simulink model "wtLinModelSimulink_LQI_V6_2021a"  (R2021a)
settings: Solver=FixedStepAuto  StartTime=0.0  StopTime=1000  FixedStep=1/25  RelTol=1e-3
values from neighbouring files (symbols this model uses):
  Alqi = [Alqr		zeros(3,1) ... (first row only)    [wtLin_V164_8MW_V6_LQI.m]
  Alqi_d = sysINT_d.A    [wtLin_V164_8MW_V6_LQI.m]
  Alqr = sysNoFLC2.A    [wtLin_V164_8MW_V6_LQI.m]
  Asys = sys.full.A    [wtLin_V164_8MW_V6_LQI.m]
  Asys_d = sys_d.A    [wtLin_V164_8MW_V6_LQI.m]
  Bdlqi = [Bdlqr; 0]    [wtLin_V164_8MW_V6_LQI.m]
  Bdlqi_d = sysINT_d.B(:,distIndex)    [wtLin_V164_8MW_V6_LQI.m]
  Bdlqr = Blqr(:, distIndex)    [wtLin_V164_8MW_V6_LQI.m]
  Bsys = sys.full.B    [wtLin_V164_8MW_V6_LQI.m]
  Bsys_d = sys_d.B    [wtLin_V164_8MW_V6_LQI.m]
  Bulqi = [Bulqr; 0]    [wtLin_V164_8MW_V6_LQI.m]
  Bulqi_d = sysINT_d.B(:,distIndex+1:end)    [wtLin_V164_8MW_V6_LQI.m]
  Bulqr = Blqr(:, distIndex+1:end)    [wtLin_V164_8MW_V6_LQI.m]
  Clqi = [Clqr	zeros(3,1)]    [wtLin_V164_8MW_V6_LQI.m]
  Clqr = sysNoFLC2.C    [wtLin_V164_8MW_V6_LQI.m]
  Csys = sys.full.C    [wtLin_V164_8MW_V6_LQI.m]
  Csys_d = sys_d.C    [wtLin_V164_8MW_V6_LQI.m]
  opWindSpeed = 16    [wtLin_V164_8MW_V6_LQI.m]
  u_op = [simulationData(1,senIdx.Vhfree); simulationData(1,senIdx.pnt413); simulationData(1,senIdx.pfo017)]    [wtLin_V164_8MW_V6_LQI.m]
  x_bar_init = [py_init vy_init W_init]'    [wtLin_V164_8MW_V6_LQI.m]
  x_bar_init_flc = [0 py_init vy_init W_init]'    [wtLin_V164_8MW_V6_LQI.m]
  x_bar_init_lqi = [py_init vy_init W_init 0]'    [wtLin_V164_8MW_V6_LQI.m]
  x_op_temp = [py_op vy_op W_op]'    [wtLin_V164_8MW_V6_LQI.m]
  x_op_temp_flc = [0 py_op vy_op W_op]'    [wtLin_V164_8MW_V6_LQI.m]
  x_op_temp_lqi = [ py_op vy_op W_op 0]'    [wtLin_V164_8MW_V6_LQI.m]
undefined symbols (not defined in the file or in its folder): Klqi, Klqi_d, Klqr2
settings Model: Creator=martin  LastModifiedBy=MROTR
settings DataIOCC: ExternalInput=tt_vfree  LoadExternalInput=on

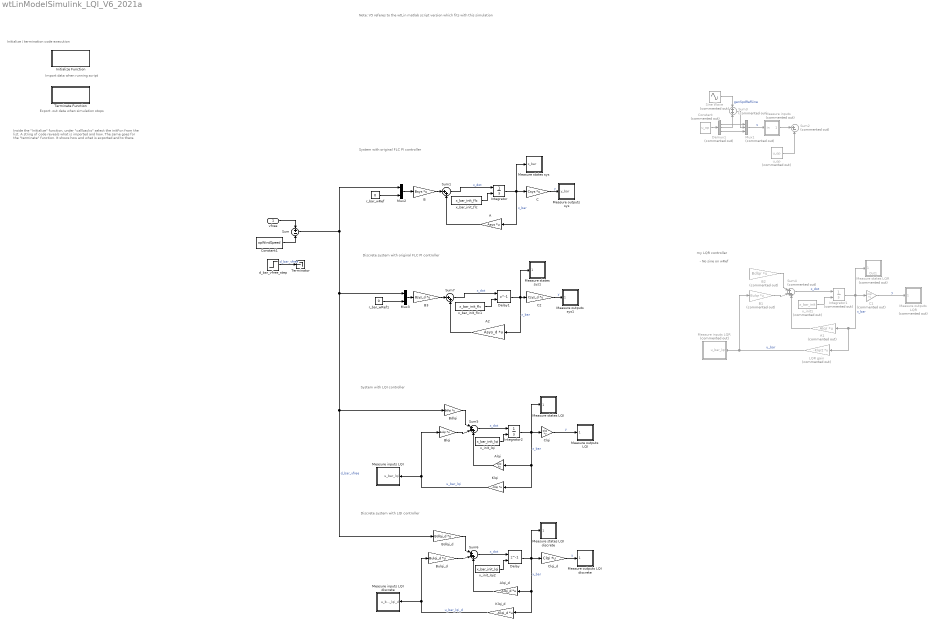
== system wtLinModelSimulink_LQI_V6_2021a ==
  note: Inside the "Initialize" function, under "callbacks" select the initFcn from the list. A string of code reveals what is imported and how.
      | The same goes for the "terminate" function. It shows how and what is exported and to there.
  note: Export .out data when simulation stops
  note: Import data when running script
  note: Initialize / termination code execution
  note: Note: V5 referes to the wtLin matlab script version which fits with this simulation
  note: System with LQI controller
  note: - No sine on wRef
  note: my LQR controller
  note: System with original FLC PI controller
  note: Discrete system with LQI controller
  note: Discrete system with original FLC PI controller
  vfree : Inport
  A : Gain  Gain=Asys  Multiplication=Matrix(K*u)
  A1 : Gain  Commented=on  Gain=Alqr  Multiplication=Matrix(K*u)
  A2 : Gain  Gain=Asys_d  Multiplication=Matrix(K*u)
  Alqi : Gain  Gain=Alqi  Multiplication=Matrix(K*u)
  Alqi_d : Gain  Gain=Alqi_d  Multiplication=Matrix(K*u)
  B : Gain  Gain=Bsys  Multiplication=Matrix(K*u)
  B1 : Gain  Commented=on  Gain=Bulqr  Multiplication=Matrix(K*u)
  B2 : Gain  Commented=on  Gain=Bdlqr  Multiplication=Matrix(K*u)
  B3 : Gain  Gain=Bsys_d  Multiplication=Matrix(K*u)
  Bdlqi : Gain  Gain=Bdlqi  Multiplication=Matrix(K*u)
  Bdlqi_d : Gain  Gain=Bdlqi_d  Multiplication=Matrix(K*u)
  Blqi : Gain  Gain=Bulqi  Multiplication=Matrix(K*u)
  Bulqi_d : Gain  Gain=Bulqi_d  Multiplication=Matrix(K*u)
  C : Gain  Gain=Csys  Multiplication=Matrix(K*u)
  C1 : Gain  Commented=on  Gain=Clqr  Multiplication=Matrix(K*u)
  C2 : Gain  Gain=Csys_d  Multiplication=Matrix(K*u)
  Clqi : Gain  Gain=Clqi  Multiplication=Matrix(K*u)
  Clqi_d : Gain  Gain=Clqi  Multiplication=Matrix(K*u)
  Constant : Constant  Commented=on  Value=u_op
  Constant1 : Constant  Value=opWindSpeed
  Delay : Delay  DelayLength=1  InitialConditionSource=Input port
      settings: InputPortMap=u0,p4
  Delay1 : Delay  DelayLength=1  InitialConditionSource=Input port
      settings: InputPortMap=u0,p4
  Demux1 : Demux  Commented=on  Outputs=3
  Initialize Function : Subsystem  InitFcn=|  TreatAsAtomicUnit=on
      | try
      |     load('c:\Users\Mrotr\Git\Repos\CA9_Project\Modelling\wtLinScriptData.mat')
      | catch exception
      |     load('/Users/martin/Documents/Git/Repos/CA9_Project/Modelling/wtLinScriptData.mat')
      | end
  Integrator : Integrator  InitialConditionSource=external
  Integrator1 : Integrator  Commented=on  InitialConditionSource=external
  Integrator2 : Integrator  InitialConditionSource=external
  Klqi : Gain  Gain=-Klqi  Multiplication=Matrix(K*u)
  Klqi_d : Gain  Gain=-Klqi_d  Multiplication=Matrix(K*u)
  LQR gain : Gain  Commented=on  Gain=-Klqr2  Multiplication=Matrix(K*u)
  Measure inputs : Subsystem  Commented=on
  Measure inputs LQI : Subsystem
  Measure inputs LQI discrete : Subsystem
  Measure inputs LQR : Subsystem  Commented=on
  Measure outputs LQI : Subsystem
  Measure outputs LQI discrete : Subsystem
  Measure outputs LQR : Subsystem  Commented=on
  Measure outputs sys : Subsystem
  Measure outputs sys1 : Subsystem
  Measure states LQI : Subsystem
  Measure states LQI discrete : Subsystem
  Measure states LQR : Subsystem  Commented=on
      settings: PortSchema="{\"entries\":[{\"content\":{\"sides\":[{\"content\":{\"connectorIds\":[\"In1\"]},\"type\":\"ConnectorPlacement.EquallySpacedRectSide\",\"uuid\":\"a5ed5e2f-8da2-4476-8dc4-f4c3a16a726d\"},{\"content\":{\"connectorIds\":[],\"side\":\"RIGHT\"},\"type\":\"ConnectorPlacement.EquallySpacedRectSide\",\"uuid\":\"b759c764-4f03-494d-936a-5a6a28e1508c\"},{\"content\":{\"connectorIds\":[],\"side\":\"TOP\"},\"type\":\"ConnectorPlacement.EquallySpacedRectSide\",\"uuid\":\"ee821022-73fd-4201-bb43-fa1eb0aa4fcb\"},{\"content\":{\"connectorIds\":[\"Out1\"],\"side\":\"BOTTOM\"},\"type\":\"ConnectorPlacement.EquallySpacedRectSide\",\"uuid\":\"2e89df74-9e94-4ecb-afc4-f716636bd492\"}]},\"type\":\"ConnectorPlacement.EquallySpacedConnector\",\"uuid\":\"bd13441d-7d6a-4a4d-915d-3d739b59ba17\"}],\"packageUris\":[\"http://schema.mathworks.com/mf0/Connector/R2020b\"],\"version\":\"1.0\"}"
  Measure states sys : Subsystem
  Measure states sys1 : Subsystem
  Mux1 : Mux  Commented=on  Inputs=3
  Mux2 : Mux  Inputs=2
  Mux3 : Mux  Inputs=2
  Sine Wave : Sin  Commented=on  Amplitude=20  Frequency=0.6302  SampleTime=0
  Sum : Sum  Inputs=+|-
  Sum1 : Sum  Inputs=|++
  Sum2 : Sum  Commented=on  Inputs=|+-
  Sum3 : Sum  Commented=on  Inputs=+|+
  Sum4 : Sum  Commented=on  Inputs=|+++
  Sum5 : Sum  Inputs=|+++
  Sum6 : Sum  Inputs=|+++
  Sum7 : Sum  Inputs=|++
  Terminate Function : Subsystem  StopFcn=|  TreatAsAtomicUnit=on
      | try
      |     save("c:\Users\Mrotr\Git\Repos\CA9_Project\Modelling\linearSimData.mat", "out")
      | catch exception
      |     save("/Users/martin/Documents/Git/Repos/CA9_Project/Modelling/linearSimData.mat", "out")
      | end
  Terminator : Terminator
  d_bar_vfree_step : Step  Time=300  After=2  SampleTime=0
  r_bar_wRef : Constant  Value=0
  r_bar_wRef1 : Constant  Value=0
  u_op : Constant  Commented=on  Value=u_op
  x_bar_init_flc : Constant  Value=x_bar_init_flc
  x_bar_init_flc1 : Constant  Value=x_bar_init_flc
  x_init1 : Constant  Commented=on  Value=x_bar_init
  x_init_lqi : Constant  Value=x_bar_init_lqi
  x_init_lqi2 : Constant  Value=x_bar_init_lqi
  wires:
  A/1 -> Sum1/2
  Sum1/1 -> Integrator/1  "x_dot"
  B/1 -> Sum1/1
  Mux1/1 -> Measure inputs/1(in)  "u"
  x_bar_init_flc/1 -> Integrator/2
  Integrator/1 -> Measure states sys/1(x_bar), C/1, A/1  "x_bar"
  Measure inputs/1(out) -> Sum2/1
  C/1 -> Measure outputs sys/1(y_bar)  "y"
  u_op/1 -> Sum2/2
  Constant/1 -> Demux1/1
  Demux1/2 -> Sum3/2
  Sine Wave/1 -> Sum3/1  "genSpdRefSine"
  Demux1/1 -> Mux1/1
  Demux1/3 -> Mux1/3
  Sum3/1 -> Mux1/2
  C1/1 -> Measure outputs LQR/1(y_bar_lqr)  "y"
  Integrator1/1 -> Measure states LQR/1(x_bar_lqr), C1/1, LQR gain/1, A1/1  "x_bar"
  A1/1 -> Sum4/3
  LQR gain/1 -> B1/1, Measure inputs LQR/1(u_bar_lqr)  "u_bar"
  x_init1/1 -> Integrator1/2
  Sum4/1 -> Integrator1/1  "x_dot"
  B1/1 -> Sum4/2
  B2/1 -> Sum4/1
  Klqi/1 -> Measure inputs LQI/1(u_bar_lqi), Blqi/1  "u_bar_lqi"
  Integrator2/1 -> Measure states LQI/1(x_bar_lqi), Clqi/1, Klqi/1, Alqi/1  "x_bar"
  x_init_lqi/1 -> Integrator2/2
  Sum5/1 -> Integrator2/1  "x_dot"
  Bdlqi/1 -> Sum5/1
  Blqi/1 -> Sum5/2
  Alqi/1 -> Sum5/3
  Clqi/1 -> Measure outputs LQI/1("y_bar_lqi ")  "y"
  r_bar_wRef/1 -> Mux2/2
  Mux2/1 -> B/1
  Constant1/1 -> Sum/2
  vfree/1 -> Sum/1
  Clqi_d/1 -> Measure outputs LQI discrete/1(y_bar_lqi_d)  "y"
  Alqi_d/1 -> Sum6/3
  Klqi_d/1 -> Measure inputs LQI discrete/1(u_bar_lqi_d), Bulqi_d/1  "u_bar_lqi_d"
  Bdlqi_d/1 -> Sum6/1
  Bulqi_d/1 -> Sum6/2
  Sum6/1 -> Delay/1  "x_dot"
  Delay/1 -> Klqi_d/1, Alqi_d/1, Measure states LQI discrete/1(x_bar_lqi_d), Clqi_d/1  "x_bar"
  x_init_lqi2/1 -> Delay/2
  B3/1 -> Sum7/1
  C2/1 -> Measure outputs sys1/1(y_bar_d)  "y"
  x_bar_init_flc1/1 -> Delay1/2
  Sum7/1 -> Delay1/1  "x_dot"
  A2/1 -> Sum7/2
  r_bar_wRef1/1 -> Mux3/2
  Delay1/1 -> Measure states sys1/1(x_bar_d), C2/1, A2/1  "x_bar"
  Mux3/1 -> B3/1
  Sum/1 -> Mux3/1, Bdlqi_d/1, Bdlqi/1, Mux2/1  "d_bar_vfree"
  d_bar_vfree_step/1 -> Terminator/1  "d_bar_vfree"

== system wtLinModelSimulink_LQI_V6_2021a/Initialize Function ==
  Event Listener : EventListener  DisableCoverage=on  EventName=reset

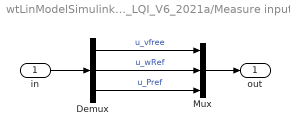
== system wtLinModelSimulink_LQI_V6_2021a/Measure inputs ==
  in : Inport
  Demux : Demux  Outputs=3
  Mux : Mux  Inputs=3
  out : Outport
  wires:
  Demux/1 -> Mux/1  "u_vfree"
  Demux/2 -> Mux/2  "u_wRef"
  Demux/3 -> Mux/3  "u_Pref"
  Mux/1 -> out/1
  in/1 -> Demux/1

== system wtLinModelSimulink_LQI_V6_2021a/Measure inputs LQI ==
  u_bar_lqi : Inport
  Derivative1 : Derivative
  Terminator2 : Terminator
  Terminator4 : Terminator
  wires:
  u_bar_lqi/1 -> Derivative1/1, Terminator2/1  "u_bar_thRef_lqi"
  Derivative1/1 -> Terminator4/1  "u_bar_thRef_deriv_lqi"

== system wtLinModelSimulink_LQI_V6_2021a/Measure inputs LQI discrete ==
  u_bar_lqi_d : Inport
  Derivative1 : Derivative
  Terminator2 : Terminator
  Terminator4 : Terminator
  wires:
  u_bar_lqi_d/1 -> Derivative1/1, Terminator2/1  "u_bar_thRef_lqi_d"
  Derivative1/1 -> Terminator4/1  "u_bar_thRef_deriv_lqi_d"

== system wtLinModelSimulink_LQI_V6_2021a/Measure inputs LQR ==
  u_bar_lqr : Inport
  Derivative1 : Derivative
  Terminator2 : Terminator
  Terminator4 : Terminator
  wires:
  u_bar_lqr/1 -> Derivative1/1, Terminator2/1  "u_bar_thRef_lqr"
  Derivative1/1 -> Terminator4/1  "u_bar_thRef_deriv_lqr"

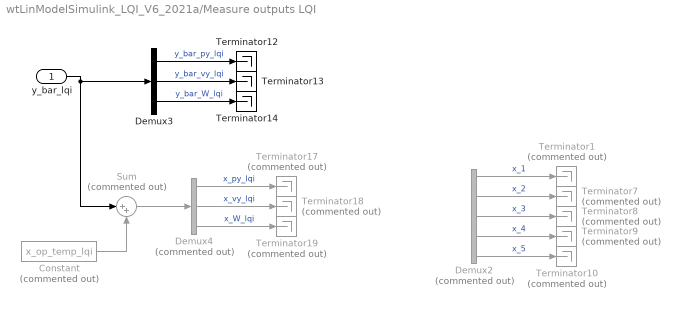
== system wtLinModelSimulink_LQI_V6_2021a/Measure outputs LQI ==
  "y_bar_lqi " : Inport
  Constant : Constant  Commented=on  Value=x_op_temp_lqi
  Demux2 : Demux  Commented=on  Outputs=5
  Demux3 : Demux  Outputs=3
  Demux4 : Demux  Commented=on  Outputs=3
  Sum : Sum  Commented=on  Inputs=|++
  Terminator{1,7..10,17..19} (8 alike) : Terminator  Commented=on
  Terminator12 : Terminator
  Terminator13 : Terminator
  Terminator14 : Terminator
  wires:
  "y_bar_lqi "/1 -> Sum/1, Demux3/1
  Constant/1 -> Sum/2
  Demux3/3 -> Terminator14/1  "y_bar_W_lqi"
  Demux3/1 -> Terminator12/1  "y_bar_py_lqi"
  Demux3/2 -> Terminator13/1  "y_bar_vy_lqi"
  Demux4/2 -> Terminator18/1  "x_vy_lqi"
  Demux4/3 -> Terminator19/1  "x_W_lqi"
  Demux4/1 -> Terminator17/1  "x_py_lqi"
  Demux2/3 -> Terminator8/1  "x_3"
  Demux2/5 -> Terminator10/1  "x_5"
  Demux2/4 -> Terminator9/1  "x_4"
  Demux2/1 -> Terminator1/1  "x_1"
  Demux2/2 -> Terminator7/1  "x_2"
  Sum/1 -> Demux4/1

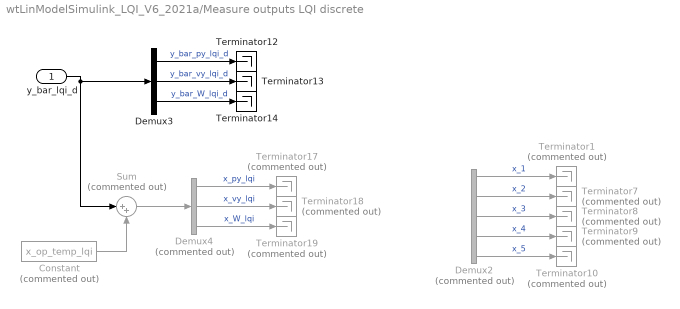
== system wtLinModelSimulink_LQI_V6_2021a/Measure outputs LQI discrete ==
  y_bar_lqi_d : Inport
  Constant : Constant  Commented=on  Value=x_op_temp_lqi
  Demux2 : Demux  Commented=on  Outputs=5
  Demux3 : Demux  Outputs=3
  Demux4 : Demux  Commented=on  Outputs=3
  Sum : Sum  Commented=on  Inputs=|++
  Terminator{1,7..10,17..19} (8 alike) : Terminator  Commented=on
  Terminator12 : Terminator
  Terminator13 : Terminator
  Terminator14 : Terminator
  wires:
  y_bar_lqi_d/1 -> Sum/1, Demux3/1
  Constant/1 -> Sum/2
  Demux3/3 -> Terminator14/1  "y_bar_W_lqi_d"
  Demux3/1 -> Terminator12/1  "y_bar_py_lqi_d"
  Demux3/2 -> Terminator13/1  "y_bar_vy_lqi_d"
  Demux4/2 -> Terminator18/1  "x_vy_lqi"
  Demux4/3 -> Terminator19/1  "x_W_lqi"
  Demux4/1 -> Terminator17/1  "x_py_lqi"
  Demux2/3 -> Terminator8/1  "x_3"
  Demux2/5 -> Terminator10/1  "x_5"
  Demux2/4 -> Terminator9/1  "x_4"
  Demux2/1 -> Terminator1/1  "x_1"
  Demux2/2 -> Terminator7/1  "x_2"
  Sum/1 -> Demux4/1

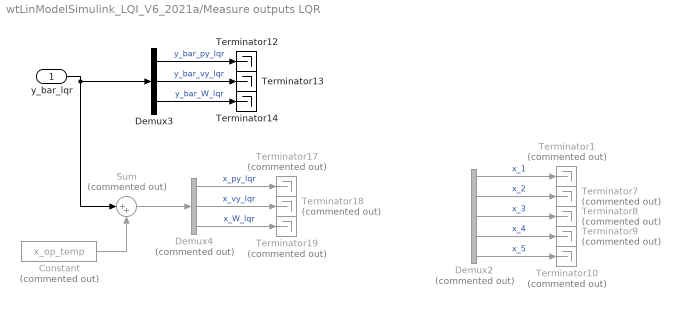
== system wtLinModelSimulink_LQI_V6_2021a/Measure outputs LQR ==
  y_bar_lqr : Inport
  Constant : Constant  Commented=on  Value=x_op_temp
  Demux2 : Demux  Commented=on  Outputs=5
  Demux3 : Demux  Outputs=3
  Demux4 : Demux  Commented=on  Outputs=3
  Sum : Sum  Commented=on  Inputs=|++
  Terminator{1,7..10,17..19} (8 alike) : Terminator  Commented=on
  Terminator12 : Terminator
  Terminator13 : Terminator
  Terminator14 : Terminator
  wires:
  y_bar_lqr/1 -> Sum/1, Demux3/1
  Constant/1 -> Sum/2
  Demux3/3 -> Terminator14/1  "y_bar_W_lqr"
  Demux3/1 -> Terminator12/1  "y_bar_py_lqr"
  Demux3/2 -> Terminator13/1  "y_bar_vy_lqr"
  Demux4/2 -> Terminator18/1  "x_vy_lqr"
  Demux4/3 -> Terminator19/1  "x_W_lqr"
  Demux4/1 -> Terminator17/1  "x_py_lqr"
  Demux2/3 -> Terminator8/1  "x_3"
  Demux2/5 -> Terminator10/1  "x_5"
  Demux2/4 -> Terminator9/1  "x_4"
  Demux2/1 -> Terminator1/1  "x_1"
  Demux2/2 -> Terminator7/1  "x_2"
  Sum/1 -> Demux4/1

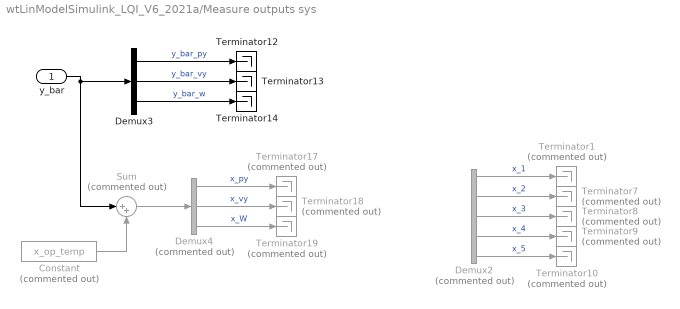
== system wtLinModelSimulink_LQI_V6_2021a/Measure outputs sys ==
  y_bar : Inport
  Constant : Constant  Commented=on  Value=x_op_temp
  Demux2 : Demux  Commented=on  Outputs=5
  Demux3 : Demux  Outputs=3
  Demux4 : Demux  Commented=on  Outputs=3
  Sum : Sum  Commented=on  Inputs=|++
  Terminator{1,7..10,17..19} (8 alike) : Terminator  Commented=on
  Terminator12 : Terminator
  Terminator13 : Terminator
  Terminator14 : Terminator
  wires:
  y_bar/1 -> Sum/1, Demux3/1
  Constant/1 -> Sum/2
  Demux3/3 -> Terminator14/1  "y_bar_w"
  Demux3/1 -> Terminator12/1  "y_bar_py"
  Demux3/2 -> Terminator13/1  "y_bar_vy"
  Demux4/2 -> Terminator18/1  "x_vy"
  Demux4/3 -> Terminator19/1  "x_W"
  Demux4/1 -> Terminator17/1  "x_py"
  Demux2/3 -> Terminator8/1  "x_3"
  Demux2/5 -> Terminator10/1  "x_5"
  Demux2/4 -> Terminator9/1  "x_4"
  Demux2/1 -> Terminator1/1  "x_1"
  Demux2/2 -> Terminator7/1  "x_2"
  Sum/1 -> Demux4/1

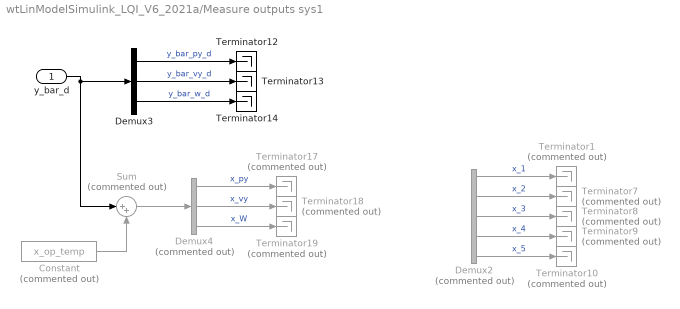
== system wtLinModelSimulink_LQI_V6_2021a/Measure outputs sys1 ==
  y_bar_d : Inport
  Constant : Constant  Commented=on  Value=x_op_temp
  Demux2 : Demux  Commented=on  Outputs=5
  Demux3 : Demux  Outputs=3
  Demux4 : Demux  Commented=on  Outputs=3
  Sum : Sum  Commented=on  Inputs=|++
  Terminator{1,7..10,17..19} (8 alike) : Terminator  Commented=on
  Terminator12 : Terminator
  Terminator13 : Terminator
  Terminator14 : Terminator
  wires:
  y_bar_d/1 -> Sum/1, Demux3/1
  Constant/1 -> Sum/2
  Demux3/3 -> Terminator14/1  "y_bar_w_d"
  Demux3/1 -> Terminator12/1  "y_bar_py_d"
  Demux3/2 -> Terminator13/1  "y_bar_vy_d"
  Demux4/2 -> Terminator18/1  "x_vy"
  Demux4/3 -> Terminator19/1  "x_W"
  Demux4/1 -> Terminator17/1  "x_py"
  Demux2/3 -> Terminator8/1  "x_3"
  Demux2/5 -> Terminator10/1  "x_5"
  Demux2/4 -> Terminator9/1  "x_4"
  Demux2/1 -> Terminator1/1  "x_1"
  Demux2/2 -> Terminator7/1  "x_2"
  Sum/1 -> Demux4/1

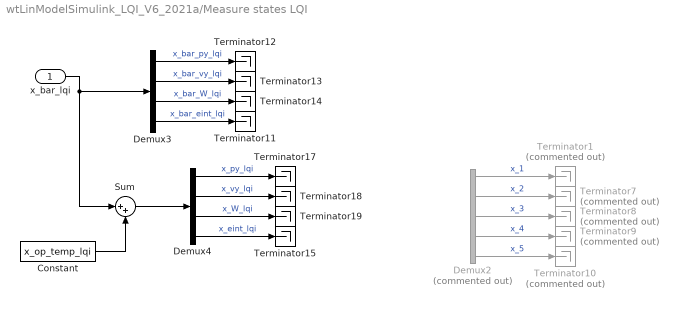
== system wtLinModelSimulink_LQI_V6_2021a/Measure states LQI ==
  x_bar_lqi : Inport
  Constant : Constant  Value=x_op_temp_lqi
  Demux2 : Demux  Commented=on  Outputs=5
  Demux3 : Demux
  Demux4 : Demux
  Sum : Sum  Inputs=|++
  Terminator{1,7..10} (5 alike) : Terminator  Commented=on
  Terminator{11..15,17..19} (8 alike) : Terminator
  wires:
  x_bar_lqi/1 -> Sum/1, Demux3/1
  Constant/1 -> Sum/2
  Demux3/3 -> Terminator14/1  "x_bar_W_lqi"
  Demux3/1 -> Terminator12/1  "x_bar_py_lqi"
  Demux3/2 -> Terminator13/1  "x_bar_vy_lqi"
  Demux4/2 -> Terminator18/1  "x_vy_lqi"
  Demux4/3 -> Terminator19/1  "x_W_lqi"
  Demux4/1 -> Terminator17/1  "x_py_lqi"
  Demux2/3 -> Terminator8/1  "x_3"
  Demux2/5 -> Terminator10/1  "x_5"
  Demux2/4 -> Terminator9/1  "x_4"
  Demux2/1 -> Terminator1/1  "x_1"
  Demux2/2 -> Terminator7/1  "x_2"
  Sum/1 -> Demux4/1
  Demux4/4 -> Terminator15/1  "x_eint_lqi"
  Demux3/4 -> Terminator11/1  "x_bar_eint_lqi"

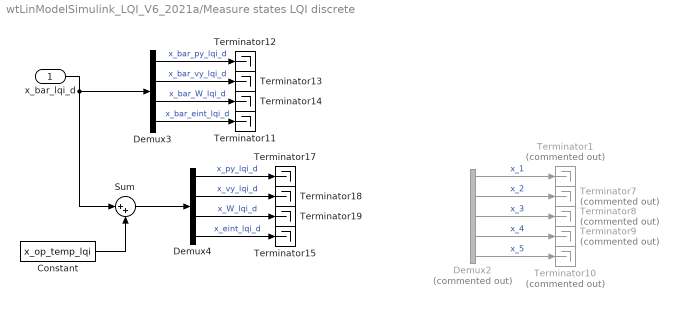
== system wtLinModelSimulink_LQI_V6_2021a/Measure states LQI discrete ==
  x_bar_lqi_d : Inport
  Constant : Constant  Value=x_op_temp_lqi
  Demux2 : Demux  Commented=on  Outputs=5
  Demux3 : Demux
  Demux4 : Demux
  Sum : Sum  Inputs=|++
  Terminator{1,7..10} (5 alike) : Terminator  Commented=on
  Terminator{11..15,17..19} (8 alike) : Terminator
  wires:
  x_bar_lqi_d/1 -> Sum/1, Demux3/1
  Constant/1 -> Sum/2
  Demux3/3 -> Terminator14/1  "x_bar_W_lqi_d"
  Demux3/1 -> Terminator12/1  "x_bar_py_lqi_d"
  Demux3/2 -> Terminator13/1  "x_bar_vy_lqi_d"
  Demux4/2 -> Terminator18/1  "x_vy_lqi_d"
  Demux4/3 -> Terminator19/1  "x_W_lqi_d"
  Demux4/1 -> Terminator17/1  "x_py_lqi_d"
  Demux2/3 -> Terminator8/1  "x_3"
  Demux2/5 -> Terminator10/1  "x_5"
  Demux2/4 -> Terminator9/1  "x_4"
  Demux2/1 -> Terminator1/1  "x_1"
  Demux2/2 -> Terminator7/1  "x_2"
  Sum/1 -> Demux4/1
  Demux4/4 -> Terminator15/1  "x_eint_lqi_d"
  Demux3/4 -> Terminator11/1  "x_bar_eint_lqi_d"

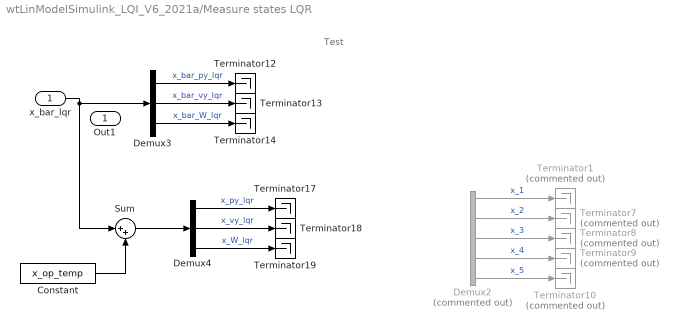
== system wtLinModelSimulink_LQI_V6_2021a/Measure states LQR ==
  note: Test
  x_bar_lqr : Inport
  Constant : Constant  Value=x_op_temp
  Demux2 : Demux  Commented=on  Outputs=5
  Demux3 : Demux  Outputs=3
  Demux4 : Demux  Outputs=3
  Sum : Sum  Inputs=|++
  Terminator{1,7..10} (5 alike) : Terminator  Commented=on
  Terminator{12..14,17..19} (6 alike) : Terminator
  Out1 : Outport
  wires:
  x_bar_lqr/1 -> Sum/1, Demux3/1
  Constant/1 -> Sum/2
  Demux3/3 -> Terminator14/1  "x_bar_W_lqr"
  Demux3/1 -> Terminator12/1  "x_bar_py_lqr"
  Demux3/2 -> Terminator13/1  "x_bar_vy_lqr"
  Demux4/2 -> Terminator18/1  "x_vy_lqr"
  Demux4/3 -> Terminator19/1  "x_W_lqr"
  Demux4/1 -> Terminator17/1  "x_py_lqr"
  Demux2/3 -> Terminator8/1  "x_3"
  Demux2/5 -> Terminator10/1  "x_5"
  Demux2/4 -> Terminator9/1  "x_4"
  Demux2/1 -> Terminator1/1  "x_1"
  Demux2/2 -> Terminator7/1  "x_2"
  Sum/1 -> Demux4/1

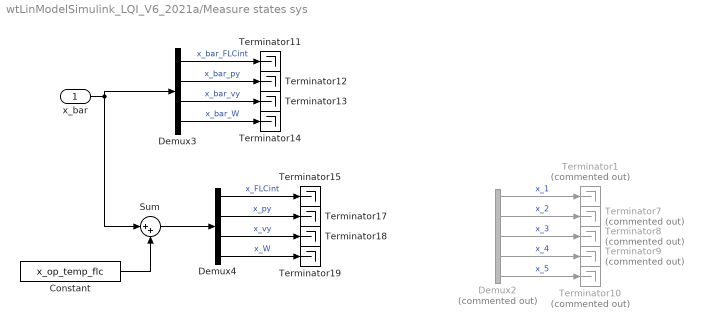
== system wtLinModelSimulink_LQI_V6_2021a/Measure states sys ==
  x_bar : Inport
  Constant : Constant  Value=x_op_temp_flc
  Demux2 : Demux  Commented=on  Outputs=5
  Demux3 : Demux
  Demux4 : Demux
  Sum : Sum  Inputs=|++
  Terminator{1,7..10} (5 alike) : Terminator  Commented=on
  Terminator{11..15,17..19} (8 alike) : Terminator
  wires:
  x_bar/1 -> Sum/1, Demux3/1
  Constant/1 -> Sum/2
  Demux3/4 -> Terminator14/1  "x_bar_W"
  Demux3/2 -> Terminator12/1  "x_bar_py"
  Demux3/3 -> Terminator13/1  "x_bar_vy"
  Demux3/1 -> Terminator11/1  "x_bar_FLCint"
  Demux4/3 -> Terminator18/1  "x_vy"
  Demux4/4 -> Terminator19/1  "x_W"
  Demux4/1 -> Terminator15/1  "x_FLCint"
  Demux4/2 -> Terminator17/1  "x_py"
  Demux2/3 -> Terminator8/1  "x_3"
  Demux2/5 -> Terminator10/1  "x_5"
  Demux2/4 -> Terminator9/1  "x_4"
  Demux2/1 -> Terminator1/1  "x_1"
  Demux2/2 -> Terminator7/1  "x_2"
  Sum/1 -> Demux4/1

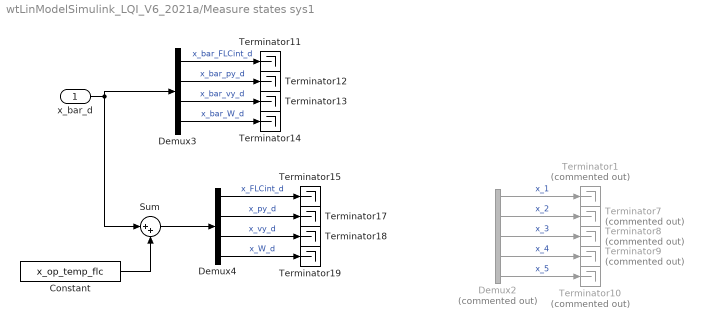
== system wtLinModelSimulink_LQI_V6_2021a/Measure states sys1 ==
  x_bar_d : Inport
  Constant : Constant  Value=x_op_temp_flc
  Demux2 : Demux  Commented=on  Outputs=5
  Demux3 : Demux
  Demux4 : Demux
  Sum : Sum  Inputs=|++
  Terminator{1,7..10} (5 alike) : Terminator  Commented=on
  Terminator{11..15,17..19} (8 alike) : Terminator
  wires:
  x_bar_d/1 -> Sum/1, Demux3/1
  Constant/1 -> Sum/2
  Demux3/4 -> Terminator14/1  "x_bar_W_d"
  Demux3/2 -> Terminator12/1  "x_bar_py_d"
  Demux3/3 -> Terminator13/1  "x_bar_vy_d"
  Demux3/1 -> Terminator11/1  "x_bar_FLCint_d"
  Demux4/3 -> Terminator18/1  "x_vy_d"
  Demux4/4 -> Terminator19/1  "x_W_d"
  Demux4/1 -> Terminator15/1  "x_FLCint_d"
  Demux4/2 -> Terminator17/1  "x_py_d"
  Demux2/3 -> Terminator8/1  "x_3"
  Demux2/5 -> Terminator10/1  "x_5"
  Demux2/4 -> Terminator9/1  "x_4"
  Demux2/1 -> Terminator1/1  "x_1"
  Demux2/2 -> Terminator7/1  "x_2"
  Sum/1 -> Demux4/1

== system wtLinModelSimulink_LQI_V6_2021a/Terminate Function ==
  Event Listener : EventListener  DisableCoverage=on  EventType=Terminate  EventName=reset
